simulink model "Model_1"  (R2019b)
settings: Solver=ode15s  StartTime=0.0  StopTime=inf  MaxStep=0.005  RelTol=1e-3
model workspace (MATLAB code in the model file):
  | ms = 135;
  | mf = 5;
  | mr = 10;
  | m = ms + (mf + mr);
  | a = 0.7;
  | b = 0.7;
  | Cd = 0.8;
  | Af = 1;
  | h_cg = 0.5;
  | kf = 10000;
  | kr = 15000;
  | cf = 5000;
  | cr = 5000;
  | I = 500;
  | kt = 175000;
values from neighbouring files (symbols this model uses):
  GR = 6.5    [Model_1_timeto40.m]    (also in Model_1_timeto60.m; Model_3_topspeed.m)
  Pmax = P(i,j)    [Model_1_timeto40.m]    (also in Model_1_timeto60.m; Model_3_topspeed.m = P(i))
  speed = 40    [Model_1_timeto40.m]    (also in Model_1_timeto60.m = 60)
  Tmax = T(i,j)    [Model_1_timeto40.m]    (also in Model_1_timeto60.m; Model_3_topspeed.m = 26)
libraries: autolibshared x2
(part 1 of 3)
settings Model: Creator=Barath Krishna S  LastModifiedBy=Barath Krishna S
settings DataIOCC: ExternalInput=[Pmax, Tmax]  SaveFormat=Array  SaveOutput=off  SaveState=on  SignalLogging=off  DSMLogging=off

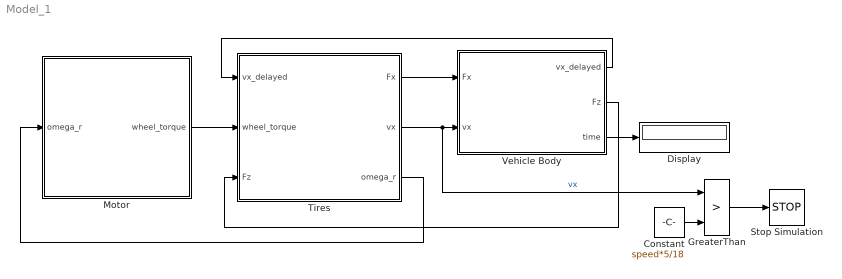
== system Model_1 ==
  Constant : Constant  Value=speed*5/18
  Display : Display
  GreaterThan : RelationalOperator  Operator=>  OutDataTypeStr=boolean  RndMeth=Simplest
  Motor : Subsystem
  Stop Simulation : Stop
  Tires : Subsystem
  Vehicle Body : Subsystem
  wires:
  Motor/1(wheel_torque) -> Tires/2(wheel_torque)
  Vehicle Body/1(vx_delayed) -> Tires/1(vx_delayed)
  Vehicle Body/2(Fz) -> Tires/3(Fz)
  Tires/2(vx) -> GreaterThan/1, Vehicle Body/2(vx)  "vx"
  Tires/1(Fx) -> Vehicle Body/1(Fx)
  Tires/3(omega_r) -> Motor/1(omega_r)
  Constant/1 -> GreaterThan/2
  GreaterThan/1 -> Stop Simulation/1
  Vehicle Body/3(time) -> Display/1

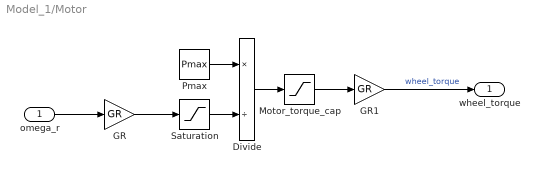
== system Model_1/Motor ==
  omega_r : Inport
  Divide : Product  Inputs=*/
  GR : Gain  Gain=GR
  GR1 : Gain  Gain=GR
  Motor_torque_cap : Saturate  UpperLimit=Tmax  LowerLimit=0
  Pmax : Constant  Value=Pmax
  Saturation : Saturate  UpperLimit=inf  LowerLimit=0.001
  wheel_torque : Outport
  wires:
  Pmax/1 -> Divide/1
  Saturation/1 -> Divide/2
  Divide/1 -> Motor_torque_cap/1
  omega_r/1 -> GR/1
  GR/1 -> Saturation/1
  Motor_torque_cap/1 -> GR1/1
  GR1/1 -> wheel_torque/1  "wheel_torque"
